simulink model "gm_cubico"  (R2017a)
settings: Solver=FixedStepDiscrete  StartTime=0.0  StopTime=10.0  FixedStep=0.001  RelTol=1e-3
undefined symbols (not defined in the file or in its folder): N
libraries: simulink x1
settings Model: Creator=Windows  LastModifiedBy=Windows
settings DataIOCC: LimitDataPoints=on  SaveOutput=off  SaveTime=off
settings OptimizationCC: BlockReduction=off  ConditionallyExecuteInputs=off  DefaultParameterBehavior=Inlined  LifeSpan=inf
settings DebuggingCC: AlgebraicLoopMsg=error  InheritedTsInSrcMsg=none  SingleTaskRateTransMsg=error  AllowSymbolicDim=off  StrictBusMsg=ErrorOnBusTreatedAsVector  SFUnexpectedBacktrackingDiag=warning  SFNoUnconditionalDefaultTransitionDiag=warning  SFExecutionAtInitializationDiag=none
settings HardwareCC: ProdBitPerPointer=32  ProdBitPerSizeT=32  ProdBitPerPtrDiffT=32  ProdLargestAtomicFloat=None  ProdIntDivRoundTo=Undefined  ProdEndianess=Unspecified  ProdWordSize=32  ProdHWDeviceType=ASIC/FPGA->ASIC/FPGA  ProdEqTarget=off
settings GRTTargetCC: TargetLangStandard=C89/C90 (ANSI)  GeneratePreprocessorConditionals=Disable all
settings ConfigComp: CovScope=ReferencedModels  CovMetricSettings=dw  CovHtmlReporting=on  CovSaveCumulativeToWorkspaceVar=on  CovSaveSingleToWorkspaceVar=on  CovExternalEMLEnable=off  CovSFcnEnable=off

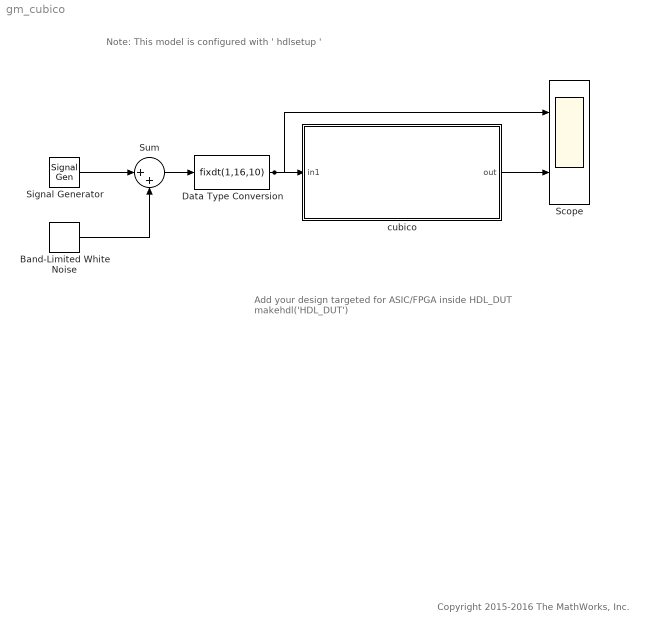
== system gm_cubico ==
  note: Copyright 2015-2016 The MathWorks, Inc.
  note: Add your design targeted for ASIC/FPGA inside HDL_DUT
      | makehdl('HDL_DUT')
  note: Note: This model is configured with ' hdlsetup '
  Band-Limited White Noise : simulink/Sources/Band-Limited White Noise  Cov=[0.001]  Ts=0.001  seed=[23341]
  Data Type Conversion : DataTypeConversion  OutDataTypeStr=fixdt(1,16,10)
  Scope : Scope  NumInputPorts=2
  Signal Generator : SignalGenerator  Frequency=2000
  Sum : Sum  Inputs=|++
  cubico : Subsystem
  wires:
  cubico/1(out) -> Scope/2
  Data Type Conversion/1 -> cubico/1(in1), Scope/1
  Band-Limited White Noise/1 -> Sum/2
  Signal Generator/1 -> Sum/1
  Sum/1 -> Data Type Conversion/1

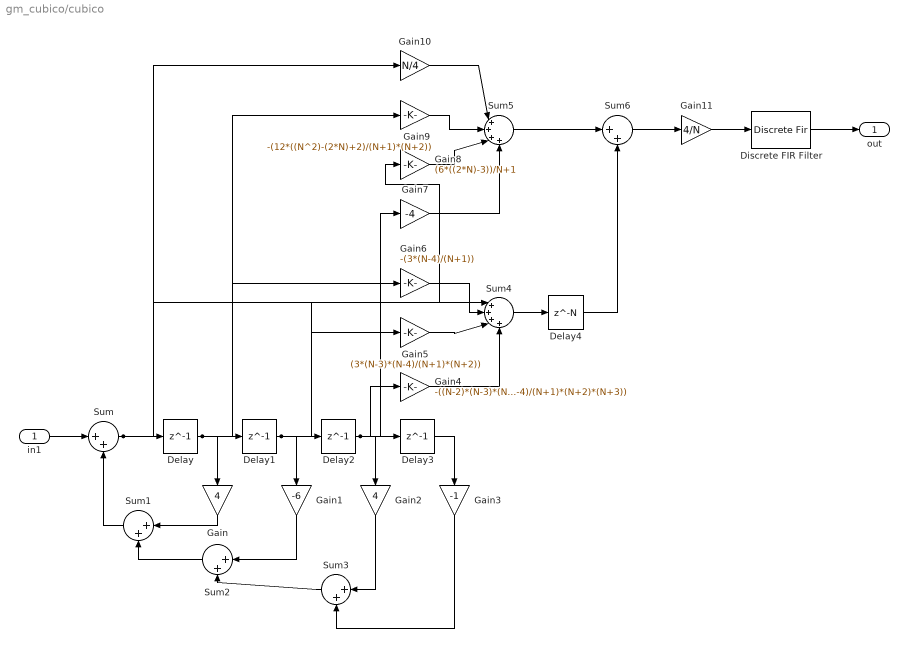
== system gm_cubico/cubico ==
  in1 : Inport  OutDataTypeStr=fixdt(1, 16, 10)  SampleTime=0
  Delay{,1..3} (4 alike) : Delay  DelayLength=1
  Delay4 : Delay  DelayLength=N
  Discrete FIR Filter : DiscreteFir  Coefficients=[0.4049 0.3288 0.2616 0.2028 0.1519 0.1085 0.0721 0.0421 0.0182 0.0008 -0.0133 -0.0220 -0.0265 -0.0274 -0.0251 -0.0201 -0.0128 -0.0038 0.0064 0.0175 0.0289 0.0402 0.0509 0.0806 0.0686 0.0747 0.0782 0.0787 0.0758 0.0690 0.0577 0.0416 0.0201 -0.0071 -0.0407]  CoefDataTypeStr=fixdt(1,16,10)  ProductDataTypeStr=fixdt(1,16,10)  AccumDataTypeStr=fixdt(1,16,10)  OutDataTypeStr=fixdt(1,16,10)
  Gain : Gain  Gain=4
  Gain1 : Gain  Gain=-6
  Gain10 : Gain  Gain=N/4
  Gain11 : Gain  Gain=4/N
  Gain2 : Gain  Gain=4
  Gain3 : Gain  Gain=-1
  Gain4 : Gain  Gain=-((N-2)*(N-3)*(N-4)/(N+1)*(N+2)*(N+3))
  Gain5 : Gain  Gain=(3*(N-3)*(N-4)/(N+1)*(N+2))
  Gain6 : Gain  Gain=-(3*(N-4)/(N+1))
  Gain7 : Gain  Gain=-4
  Gain8 : Gain  Gain=(6*((2*N)-3))/N+1
  Gain9 : Gain  Gain=-(12*((N^2)-(2*N)+2)/(N+1)*(N+2))
  Sum{,1..3,6} (5 alike) : Sum  Inputs=|++  AccumDataTypeStr=fixdt(1,16,10)  OutDataTypeStr=fixdt(1,16,10)
  Sum4 : Sum  Inputs=|++++  AccumDataTypeStr=fixdt(1,16,10)  OutDataTypeStr=fixdt(1,16,10)
  Sum5 : Sum  Inputs=|++++  AccumDataTypeStr=fixdt(1,16,10)  OutDataTypeStr=fixdt(1,16,10)
  out : Outport  OutDataTypeStr=fixdt(1,16,10)
  wires:
  in1/1 -> Sum/1
  Delay/1 -> Gain9/1, Gain6/1, Gain/1, Delay1/1
  Delay1/1 -> Gain8/1, Gain5/1, Gain1/1, Delay2/1
  Delay2/1 -> Gain7/1, Gain4/1, Gain2/1, Delay3/1
  Delay3/1 -> Gain3/1
  Delay4/1 -> Sum6/2
  Discrete FIR Filter/1 -> out/1
  Gain/1 -> Sum1/1
  Gain1/1 -> Sum2/1
  Gain10/1 -> Sum5/1
  Gain11/1 -> Discrete FIR Filter/1
  Gain2/1 -> Sum3/1
  Gain3/1 -> Sum3/2
  Gain4/1 -> Sum4/4
  Gain5/1 -> Sum4/3
  Gain6/1 -> Sum4/2
  Gain7/1 -> Sum5/4
  Gain8/1 -> Sum5/3
  Gain9/1 -> Sum5/2
  Sum/1 -> Sum4/1, Gain10/1, Delay/1
  Sum1/1 -> Sum/2
  Sum2/1 -> Sum1/2
  Sum3/1 -> Sum2/2
  Sum4/1 -> Delay4/1
  Sum5/1 -> Sum6/1
  Sum6/1 -> Gain11/1
